simulink model "project_model_lqi_Matlab2017"  (R2021a)
settings: Solver=FixedStepDiscrete  StartTime=0.0  StopTime=450  FixedStep=0.5  MaxStep=1  RelTol=1e-3
undefined symbols (not defined in the file or in its folder): DiscIntNeverNeededParam, Discrete, Time
libraries: ctrlSharedLib x1
settings Model: Creator=Admin  LastModifiedBy=click
settings SolverCC: AlgebraicLoopSolver=TrustRegion
settings DataIOCC: ReturnWorkspaceOutputs=off
settings DebuggingCC: SFMachineParentedDataDiag=warning  ArithmeticOperatorsInVariantConditions=warning
settings SFSimCC: SimUseLocalCustomCode=off  CustomCodeUndefinedFunction=UseInterfaceOnly
settings RTWCC: RTWUseLocalCustomCode=off
settings CodeAppCC: StateflowObjectComments=on

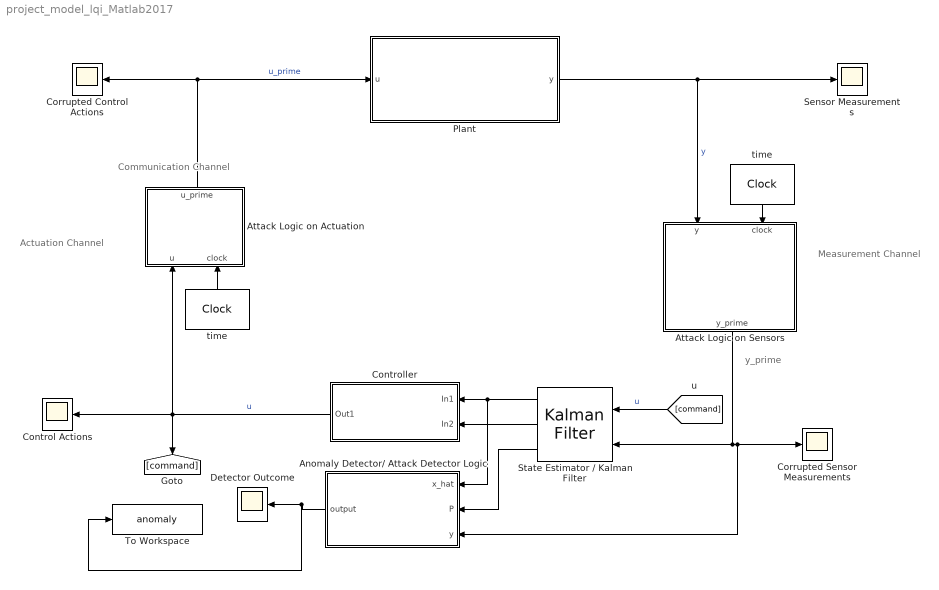
== system project_model_lqi_Matlab2017 ==
  note: y_prime
  note: Communication Channel
  note: Measurement Channel
  note: Actuation Channel
  Anomaly Detector/ Attack Detector Logic : MATLAB Function  TreatAsAtomicUnit=on
  Attack Logic on Actuation : MATLAB Function  TreatAsAtomicUnit=on
  Attack Logic on Sensors : MATLAB Function  TreatAsAtomicUnit=on
  Control Actions : Scope
  Controller : Subsystem
  Corrupted Control Actions : Scope
  Corrupted Sensor Measurements : Scope
  Detector Outcome : Scope
  Plant : Subsystem
  "Sensor Measurements " : Scope
  State Estimator / Kalman Filter : ctrlSharedLib/Kalman Filter  TimeDomain=Discrete-Time  UseCurrentEstimator=off  ModelSource=Individual A, B, C, D matrices  ModelSourceVariable=sys  A="[0.9719  -0.0013;-0.0340  0.8628]"  B="[-0.0839  0.0232;0.0761  0.4144]"  C=[0 1]  D=0  NumberOfStates=2  NumberOfInputs=2  NumberOfOutputs=2  InitialEstimateSource=Dialog  X0=[0]  P0=10  UseK=off  UseGH=off  NumberOfProcessNoiseInputs=2  G=B  TimeInvariantG=on  H=0  TimeInvariantH=on  Q=0.001*eye(2)  TimeInvariantQ=on  R=0.01  TimeInvariantR=on  N=0  TimeInvariantN=on  AddInputPort=on  AddEnablePort=off  OutputEstimatedY=on  OutputP=on  Ts=0.5
  To Workspace : ToWorkspace  VariableName=anomaly  SampleTime=-1
      settings: Save2DSignal=2-D array (concatenate along first dimension)
  time : DigitalClock  SampleTime=0.5
  "time " : DigitalClock  SampleTime=0.5
  wires:
  Anomaly Detector/ Attack Detector Logic/1(output) -> To Workspace/1, Detector Outcome/1
  "time "/1 -> Attack Logic on Sensors/2(clock)
  Attack Logic on Sensors/1(y_prime) -> Corrupted Sensor Measurements/1, Anomaly Detector/ Attack Detector Logic/3(y), State Estimator / Kalman Filter/2
  Controller/1(Out1) -> [command], Control Actions/1, Attack Logic on Actuation/1(u)  "u"
  time/1 -> Attack Logic on Actuation/2(clock)
  Attack Logic on Actuation/1(u_prime) -> Corrupted Control Actions/1, Plant/1(u)  "u_prime"
  Plant/1(y) -> Attack Logic on Sensors/1(y), "Sensor Measurements "/1  "y"
  State Estimator / Kalman Filter/1 -> Anomaly Detector/ Attack Detector Logic/1(x_hat), Controller/1(In1)
  State Estimator / Kalman Filter/3 -> Anomaly Detector/ Attack Detector Logic/2(P)
  State Estimator / Kalman Filter/2 -> Controller/2(In2)
  [command] -> State Estimator / Kalman Filter/1  "u"

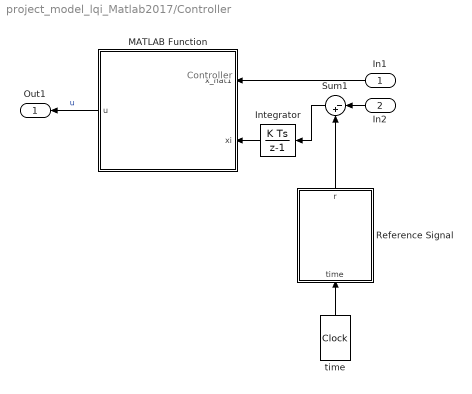
== system project_model_lqi_Matlab2017/Controller ==
  note: Controller
  In1 : Inport
  In2 : Inport  Port=2
  Integrator : DiscreteIntegrator  SampleTime=0.5  ICPrevOutput=DiscIntNeverNeededParam  ICPrevScaledInput=DiscIntNeverNeededParam
  MATLAB Function : MATLAB Function  TreatAsAtomicUnit=on
  Reference Signal : MATLAB Function  TreatAsAtomicUnit=on
  Sum1 : Sum  Inputs=|-+
  "time   " : DigitalClock  SampleTime=0.5
  Out1 : Outport
  wires:
  Sum1/1 -> Integrator/1
  In1/1 -> MATLAB Function/1(x_hat1)
  MATLAB Function/1(u) -> Out1/1  "u"
  In2/1 -> Sum1/1
  Integrator/1 -> MATLAB Function/2(xi)
  Reference Signal/1(r) -> Sum1/2
  "time   "/1 -> Reference Signal/1(time)

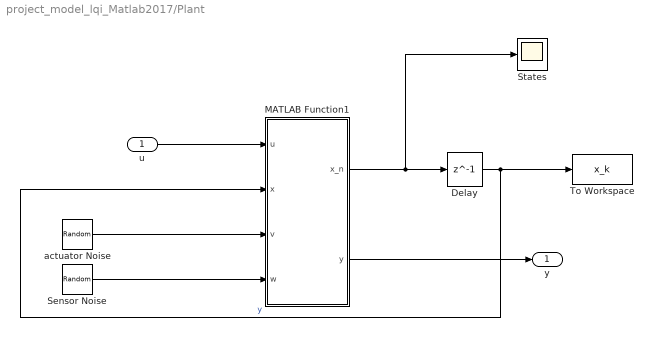
== system project_model_lqi_Matlab2017/Plant ==
  u : Inport
  Delay : Delay  DelayLength=1  InitialCondition=[0 0]  SampleTime=0.5
  MATLAB Function1 : MATLAB Function  TreatAsAtomicUnit=on
  Sensor Noise : RandomNumber  Mean=[0]  Variance=[0.01]  Seed=[randi(100)]  SampleTime=0.5
  States : Scope
  To Workspace : ToWorkspace  VariableName=x_k  SaveFormat=Timeseries  SampleTime=-1
  actuator Noise : RandomNumber  Mean=[0 0]  Variance=[0.001 0.001]  Seed=[randi(100) randi(100)]  SampleTime=0.5
  y : Outport
  wires:
  u/1 -> MATLAB Function1/1(u)
  MATLAB Function1/1(x_n) -> States/1, Delay/1
  MATLAB Function1/2(y) -> y/1
  Delay/1 -> To Workspace/1, MATLAB Function1/2(x)  "y"
  actuator Noise/1 -> MATLAB Function1/3(v)
  Sensor Noise/1 -> MATLAB Function1/4(w)

== matlab function project_model_lqi_Matlab2017/Attack Logic on Sensors ==
  data: y input; y_prime output; clock input
function y_prime = fcn(y,clock)
% this function should contain the attacker action on the sensor
% measurements

y_prime=y;


end

== matlab function project_model_lqi_Matlab2017/Controller/MATLAB Function ==
  data: x_hat1 input; u output; xi input
function u  = Controller(x_hat1,xi)
    
x=[x_hat1;xi];
%controller gain
% K=[-22.0702    1.2177   -0.0582
%     4.0113    4.3249   -0.3108];

K= [-0.7037, 0.2666, -0.1324
   0.0535,1.3382,-0.7004];


u=-K*x;

== matlab function project_model_lqi_Matlab2017/Attack Logic on Actuation ==
  data: u input; u_prime output; clock input
function u_prime = fcn(u,clock)
% this function should contain the attacker action on the control inputs
uacutator = [0;0];
if (clock >= 0 && clock < 50)

   uacutator = [0;0];
   

   elseif (clock >= 50 && clock  < 250)

   uacutator = [clock/250; clock/250];
   
   
    
   elseif (clock >= 250 && clock  < 450)
  
   uacutator = [clock/900; clock/900];
      
    

   elseif (clock >= 450) 

     uacutator = [0;0];


 end
      u_prime = u+uacutator ;

end

== matlab function project_model_lqi_Matlab2017/Anomaly Detector// Attack Detector Logic ==
  data: x_hat input; output output; P input; y input
function output  = Detector(x_hat,P, y)
% this function should contain the detection strategy



alpha = 0.08;
v = 1;
C = [0,1];
R = 0.01;

%chi square is calculated here

tau = chi2inv(1-alpha,v);
r = y-(C*x_hat);
sigma = (C*P*(transpose(C)))+ R;
z = transpose(r)*(inv(sigma))*r;
chi = z;


if chi <= tau
    %disp('no alarm');
    attack = 0;
    
else
    %disp('alarm');
    attack = 1;
end

output = attack;
end

== matlab function project_model_lqi_Matlab2017/Plant/MATLAB Function1 ==
  data: x_n output; u input; y output; x input; v input; w input
function [x_n, y] = fcn(u, x, v, w)

A=[	0.9719  -0.0013;-0.0340  0.8628];
B=[-0.0839  0.0232;0.0761  0.4144];
C=[0 1];
D=[0 0];

x_n = A*x + B*u + v;
y = C*x + D*u + w;

== matlab function project_model_lqi_Matlab2017/Controller/Reference Signal ==
  data: r output; time input
function r = fcn(time)
%#codegen
r=[0];
if time < 100
    r=[0];
elseif 100<=time && time<350
    r=[8];
elseif 350<=time
    r=[-5];
end
